simulink model "Armonicos"  (R2017b)
settings: Solver=VariableStepDiscrete  StartTime=0.0  StopTime=1/60*5  MaxStep=1e-4  RelTol=1e-3
libraries: powerlib x10, powerlib_meascontrol x2
settings Model: Creator=DiegoUlises  LastModifiedBy=DiegoUlises

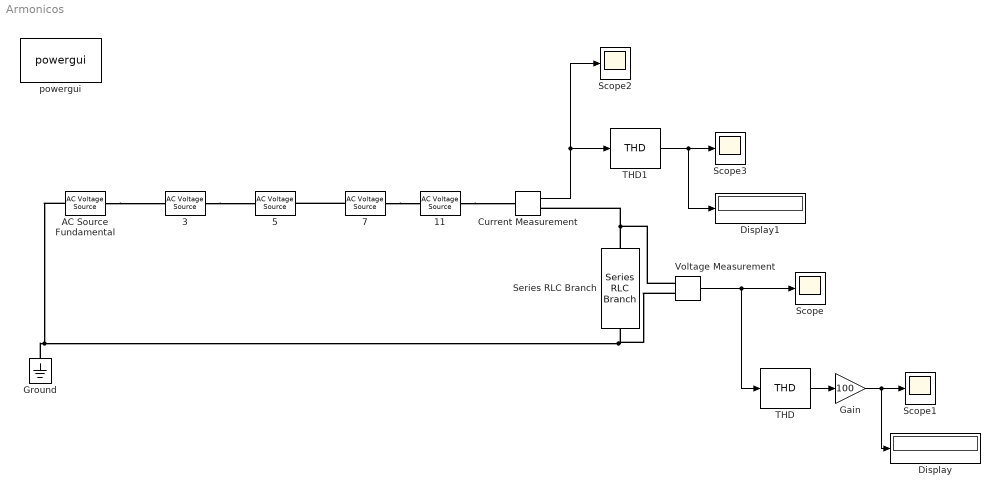
== system Armonicos ==
  11 : powerlib/Electrical Sources/AC Voltage Source  Amplitude=10  Phase=0  Frequency=60*11  SampleTime=1e-6  Measurements=None  BusType=swing  Pref=10e3  Qref=0  Qmin=-inf  Qmax=+inf
  "3 " : powerlib/Electrical Sources/AC Voltage Source  Amplitude=80  Phase=0  Frequency=60*3  SampleTime=1e-6  Measurements=None  BusType=swing  Pref=10e3  Qref=0  Qmin=-inf  Qmax=+inf
  "5 " : powerlib/Electrical Sources/AC Voltage Source  Amplitude=50  Phase=0  Frequency=60*5  SampleTime=1e-6  Measurements=None  BusType=swing  Pref=10e3  Qref=0  Qmin=-inf  Qmax=+inf
  "7 " : powerlib/Electrical Sources/AC Voltage Source  Amplitude=30  Phase=0  Frequency=60*7  SampleTime=1e-6  Measurements=None  BusType=swing  Pref=10e3  Qref=0  Qmin=-inf  Qmax=+inf
  AC Source Fundamental : powerlib/Electrical Sources/AC Voltage Source  Amplitude=140  Phase=0  Frequency=60  SampleTime=1e-6  Measurements=None  BusType=swing  Pref=10e3  Qref=0  Qmin=-inf  Qmax=+inf
  "Current Measurement " : powerlib/Measurements/Current Measurement  PhasorSimulation=off  OutputType=Complex  PSBequivalent=0
  "Display " : Display
  "Display1 " : Display
  "Gain " : Gain  Gain=100
  Ground : powerlib/Elements/Ground  LConnTagsString=a
  "Scope " : Scope
  "Scope1 " : Scope
  "Scope2 " : Scope
  "Scope3 " : Scope
  Series RLC Branch : powerlib/Elements/Series RLC Branch  LConnTagsString=__new0  RConnTagsString=__new0  BranchType=R  Resistance=1  Inductance=1e-3  SetiL0=off  InitialCurrent=0  Capacitance=1e-6  Setx0=off  InitialVoltage=0  Measurements=None
  "THD " : powerlib_meascontrol/Measurements/THD  Freq=60  Ts=1e-6
  "THD1 " : powerlib_meascontrol/Measurements/THD  Freq=60  Ts=1e-6
  Voltage Measurement : powerlib/Measurements/Voltage Measurement  PhasorSimulation=off  OutputType=Complex  PSBequivalent=0
  powergui : powerlib/powergui  Priority=1  SimulationMode=Discrete  SampleTime=1e-6  frequency=60  Iterations=50  frequencyindice=60  Pbase=100e6  ErrMax=1e-4  UnitsV=kV  UnitsW=MW  buscounter=0  FunctionMessages=off  echomessages=off  EnableUseOfTLC=off  CurrentSourceSwitches=off  DisableSnubberDevices=off  DisableRonSwitches=off  DisableVfSwitches=off  DisplayEquations=off  SolverType=Tustin/Backward Euler (TBE)  Interpol=off  ExternalGateDelay=off  methode=off  Ts=100  x0status=blocks  SPID=on  SwTol=0  HookPort=off  RestoreLinks=warning  ResistiveCurrentMeasurement=off  Frange=[0:2:500]  Ylog=off  Xlog=on  ShowGrid=off  save=off  variable=ZData  structure=0  ZoomFFT=off  StartTime=0.0  cycles=1  DisplayStyle=1  fundamental=60  FreqAxis=off  MaxFrequency=1000  frequencyindicesteady=1  RmsSteady=1  display=off
  wires:
  Voltage Measurement/1 -> "THD "/1, "Scope "/1
  "THD "/1 -> "Gain "/1
  "Gain "/1 -> "Display "/1, "Scope1 "/1
  "Current Measurement "/1 -> "THD1 "/1, "Scope2 "/1
  "THD1 "/1 -> "Display1 "/1, "Scope3 "/1
  connections:
  "7 "/LConn1 -- "5 "/RConn1
  Series RLC Branch/LConn1 -- Voltage Measurement/LConn1 -- "Current Measurement "/RConn1
  AC Source Fundamental/LConn1 -- Voltage Measurement/LConn2 -- Series RLC Branch/RConn1 -- Ground/LConn1
  AC Source Fundamental/RConn1 -- "3 "/LConn1
  "3 "/RConn1 -- "5 "/LConn1
  "7 "/RConn1 -- 11/LConn1
  11/RConn1 -- "Current Measurement "/LConn1
